simulink model "test_model"  (R2023a)
settings: Solver=VariableStepAuto  StartTime=0.0  StopTime=10.0  RelTol=1e-3
undefined symbols (not defined in the file): x
settings Model: Creator=ayind  LastModifiedBy=ayind

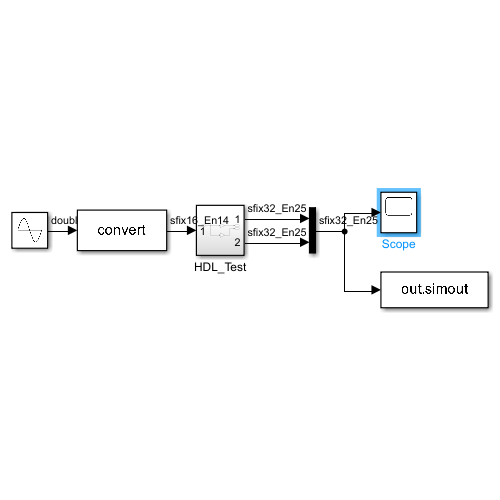
[thumbnail: Simulink's stored preview of the top-level diagram]
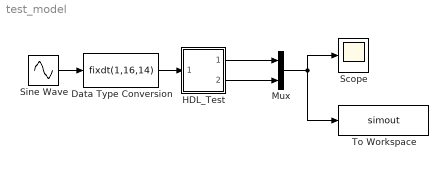
== system test_model ==
  Data Type Conversion : DataTypeConversion  OutDataTypeStr=fixdt(1,16,14)  SaturateOnIntegerOverflow=off  RndMeth=Floor
  HDL_Test : Subsystem
  Mux : Mux  Inputs=2
  Scope : Scope
  Sine Wave : Sin  SampleTime=0
  To Workspace : ToWorkspace  VariableName=simout  SaveFormat=Timeseries  SampleTime=-1
  wires:
  Mux/1 -> To Workspace/1, Scope/1
  Sine Wave/1 -> Data Type Conversion/1
  HDL_Test/1(Out1) -> Mux/1
  HDL_Test/2(Out2) -> Mux/2
  Data Type Conversion/1 -> HDL_Test/1(In1)

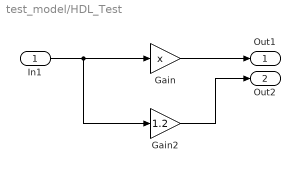
== system test_model/HDL_Test ==
  In1 : Inport
  Gain : Gain  Gain=x  OutDataTypeStr=fixdt(1,32,25)
  Gain2 : Gain  Gain=1.2  OutDataTypeStr=fixdt(1,32,25)
  Out1 : Outport
  Out2 : Outport  Port=2
  wires:
  In1/1 -> Gain2/1, Gain/1
  Gain2/1 -> Out2/1
  Gain/1 -> Out1/1
